simulink model "emgSubscriber"  (R2017a)
settings: Solver=VariableStepAuto  StartTime=0.0  StopTime=inf  FixedStep=0.004  RelTol=1e-3
undefined symbols (not defined in the file or in its folder): A_butter_cal, B_butter_cal
libraries: robotlib x1
settings Model: Creator=jacob  LastModifiedBy=jacob

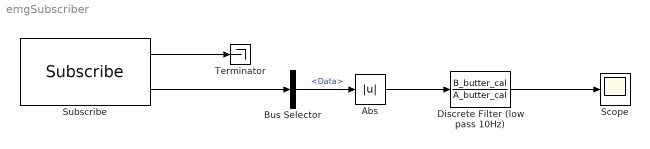
== system emgSubscriber ==
  Abs : Abs
  Bus Selector : BusSelector  OutputSignals=Data
  Discrete Filter (low pass 10Hz) : DiscreteFilter  Numerator=B_butter_cal  Denominator=A_butter_cal
  Scope : Scope
  Subscribe : robotlib/Subscribe  SourceLibraryInfo=This block requires Robotics System Toolbox  topicSource=Select from ROS network  topic=/emgPub  messageType=std_msgs/Int64  sampleTime=-1  messageQueueLength=1
      settings: SourceProductBaseCode=RO
  Terminator : Terminator
  wires:
  Subscribe/1 -> Terminator/1
  Subscribe/2 -> Bus Selector/1
  Bus Selector/1 -> Abs/1  "<Data>"
  Abs/1 -> Discrete Filter (low pass 10Hz)/1
  Discrete Filter (low pass 10Hz)/1 -> Scope/1
